simulink model "untitled1"  (R2024b)
settings: Solver=VariableStepAuto  StartTime=0.0  StopTime=10  RelTol=1e-3
libraries: vrlib x1
settings Model: PacingRate=0.100000  Creator=mattia  LastModifiedBy=mattia

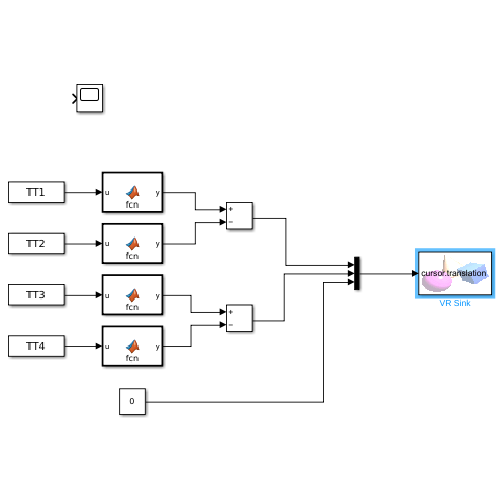
[thumbnail: Simulink's stored preview of the top-level diagram]
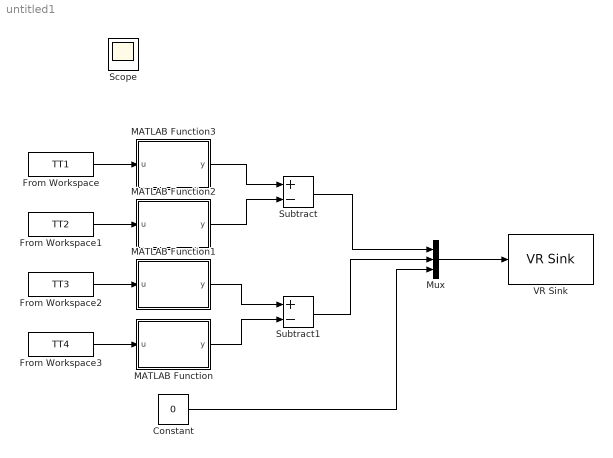
== system untitled1 ==
  Constant : Constant  Value=0
  From Workspace : FromWorkspace  VariableName=TT1
  From Workspace1 : FromWorkspace  VariableName=TT2
  From Workspace2 : FromWorkspace  VariableName=TT3
  From Workspace3 : FromWorkspace  VariableName=TT4
  MATLAB Function : MATLAB Function  TreatAsAtomicUnit=on
  MATLAB Function1 : MATLAB Function  TreatAsAtomicUnit=on
  MATLAB Function2 : MATLAB Function  TreatAsAtomicUnit=on
  MATLAB Function3 : MATLAB Function  TreatAsAtomicUnit=on
  Mux : Mux  Inputs=3
  Scope : Scope
  Subtract : Sum  Inputs=+-
  Subtract1 : Sum  Inputs=+-
  VR Sink : vrlib/VR Sink  InstantiateOnLoad=on  SampleTime=0.1  ViewEnable=on  RemoteChange=off  RemoteView=off  FieldsWritten=cursor.translation.3.1.1.double  WorldFileName=8_palline_color.wrl  AutoView=off  VideoDimensions=[]  AllowVariableSize=off
  wires:
  Mux/1 -> VR Sink/1
  Constant/1 -> Mux/3
  From Workspace/1 -> MATLAB Function3/1(u)
  MATLAB Function3/1(y) -> Subtract/1
  MATLAB Function2/1(y) -> Subtract/2
  Subtract/1 -> Mux/1
  MATLAB Function1/1(y) -> Subtract1/1
  MATLAB Function/1(y) -> Subtract1/2
  Subtract1/1 -> Mux/2
  From Workspace1/1 -> MATLAB Function2/1(u)
  From Workspace2/1 -> MATLAB Function1/1(u)
  From Workspace3/1 -> MATLAB Function/1(u)

== matlab function untitled1/MATLAB Function ==
  data: u input; y output
function y = fcn(u)

val = u*0.1/0.22;

if val > 0.1 
    y = 0.1;
elseif val > 0.01
    y = val;
else 
    y = 0;
end

== matlab function untitled1/MATLAB Function2 ==
  data: u input; y output
function y = fcn(u)

val = u*0.1/0.008;

if val > 0.1 
    y = 0.1;
elseif val > 0.01
    y = val;
else 
    y = 0;
end

== matlab function untitled1/MATLAB Function3 ==
  data: u input; y output
function y = fcn(u)

val = u*0.1/0.4;

if val > 0.1 
    y = 0.1;
elseif val > 0.01
    y = val;
else 
    y = 0;
end

== matlab function untitled1/MATLAB Function1 ==
  data: u input; y output
function y = fcn(u)

val = u*0.1/0.2;

if val > 0.1 
    y = 0.1;
elseif val > 0.01
    y = val;
else 
    y = 0;
end
